simulink model "Lab1_simulink"  (R2024b)
settings: Solver=VariableStepAuto  StartTime=0.0  StopTime=10000  MaxStep=0.1  RelTol=1e-3
values from neighbouring files (symbols this model uses):
  Gb = 81    [parametri.m]
  Ib = 15    [parametri.m]
  n = 5/54    (= 0.0925925925926)    [parametri.m]
  p1 = 0.003    [parametri.m]
  p2 = 0.025    [parametri.m]
  p3 = 0.000013    (= 1.3e-05)    [parametri.m]
  r = 16.66667    [parametri.m]
  V1 = 12    [parametri.m]
  Vg = 126    [parametri.m]
libraries: simulink x4
settings Model: Creator=stefa  LastModifiedBy=stefa
settings RTWCC: GPUComputeCapability=3.5
settings GRTTargetCC: RTWCAPISignals=on  RTWCAPIParams=on

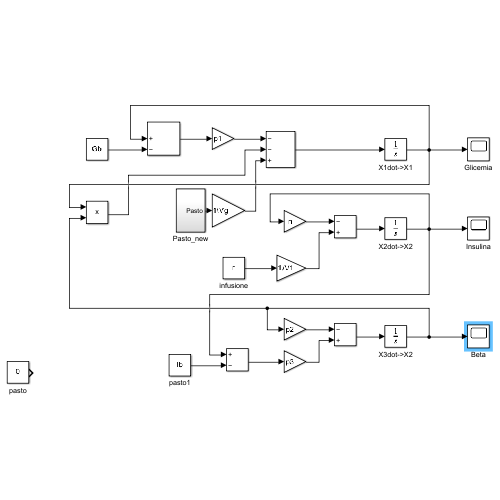
[thumbnail: Simulink's stored preview of the top-level diagram]
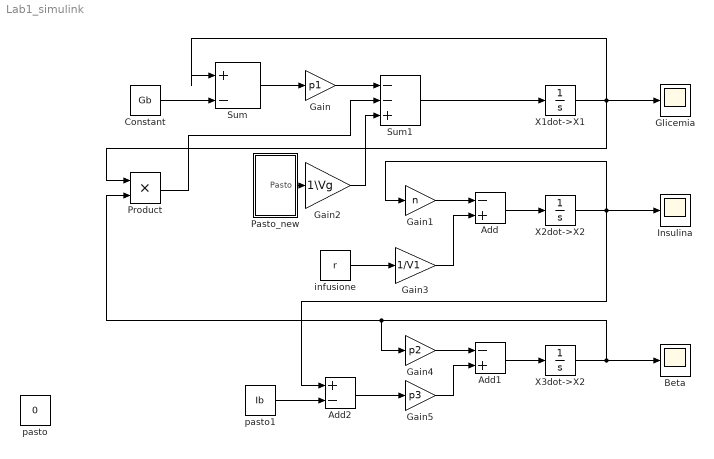
== system Lab1_simulink ==
  Add : Sum  Inputs=-+
  Add1 : Sum  Inputs=-+
  Add2 : Sum  Inputs=+-
  Beta : Scope
  Constant : Constant  Value=Gb
  Gain : Gain  Gain=p1
  Gain1 : Gain  Gain=n
  Gain2 : Gain  Gain=1\Vg
  Gain3 : Gain  Gain=1/V1
  Gain4 : Gain  Gain=p2
  Gain5 : Gain  Gain=p3
  Glicemia : Scope
  Insulina : Scope
  Pasto_new : Subsystem
  Product : Product
  Sum : Sum  Inputs=|+-
  Sum1 : Sum  Inputs=--+
  X1dot->X1 : Integrator
  X2dot->X2 : Integrator
  X3dot->X2 : Integrator
  infusione : Constant  Value=r
  pasto : Constant  Value=0
  pasto1 : Constant  Value=Ib
  wires:
  Constant/1 -> Sum/2
  X1dot->X1/1 -> Sum/1, Product/1, Glicemia/1
  Sum/1 -> Gain/1
  Gain/1 -> Sum1/1
  Product/1 -> Sum1/2
  X3dot->X2/1 -> Gain4/1, Product/2, Beta/1
  Gain2/1 -> Sum1/3
  Sum1/1 -> X1dot->X1/1
  Add/1 -> X2dot->X2/1
  Gain1/1 -> Add/1
  X2dot->X2/1 -> Gain1/1, Add2/1, Insulina/1
  Gain3/1 -> Add/2
  infusione/1 -> Gain3/1
  Gain4/1 -> Add1/1
  Add1/1 -> X3dot->X2/1
  Gain5/1 -> Add1/2
  Add2/1 -> Gain5/1
  pasto1/1 -> Add2/2
  Pasto_new/1(Pasto) -> Gain2/1

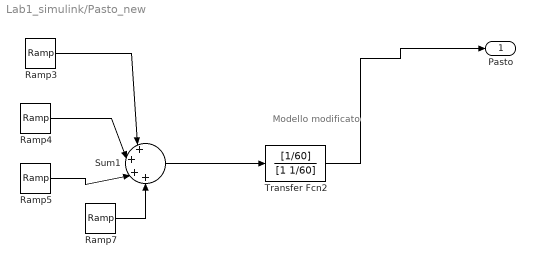
== system Lab1_simulink/Pasto_new ==
  note: Modello
      | modificato
  Ramp3 : simulink/Sources/Ramp  slope=12  start=0  InitialOutput=0
  Ramp4 : simulink/Sources/Ramp  slope=-12  start=30  InitialOutput=0
  Ramp5 : simulink/Sources/Ramp  slope=-12  start=90  InitialOutput=0
  Ramp7 : simulink/Sources/Ramp  slope=12  start=120  InitialOutput=0
  Sum1 : Sum  Inputs=|+|+|+|+  InputSameDT=on  SaturateOnIntegerOverflow=on  OutDataTypeStr=Inherit: Same as first input
  Transfer Fcn2 : TransferFcn  Numerator=[1/60]  Denominator=[1 1/60]
  Pasto : Outport
  wires:
  Ramp3/1 -> Sum1/1
  Ramp4/1 -> Sum1/2
  Ramp5/1 -> Sum1/3
  Ramp7/1 -> Sum1/4
  Sum1/1 -> Transfer Fcn2/1
  Transfer Fcn2/1 -> Pasto/1
